simulink model "Drone_PID_rev5_Manual_PID_RL"  (R2021b)
settings: Solver=ode5  StartTime=0.0  StopTime=60  FixedStep=1e-2  RelTol=1e-3
values from neighbouring files (symbols this model uses):
  g = robot.env.g    [A_Main.m]
  Kf = robot.aero.Kthrust    [A_Main.m]
  Km = robot.aero.Ktorque    [A_Main.m]
  L = robot.geom.L    [A_Main.m]
  mass = robot.geom.mass*(0.40*rand()-0.20+1)    [A_Main.m]
  maxRPM = robot.rotor.rpm    [A_Main.m]
  T = [Kf                              Kf                             Kf                             Kf ... (first row only)    [A_Main.m]
  Tinv = inv(T)    [A_Main.m]
  Wmax = maxRPM*2*pi/60    [A_Main.m]
undefined symbols (not defined in the file or in its folder): DiscIntNeverNeededParam, sigbuilder_block
libraries: simulink x16, aerolibconvert2 x13, rllib x4, shared6dof x1
settings Model: Creator=Hassan  LastModifiedBy=Hassan
settings SolverCC: AlgebraicLoopSolver=TrustRegion
settings DebuggingCC: ArithmeticOperatorsInVariantConditions=warning
settings SFSimCC: CustomCodeUndefinedFunction=UseInterfaceOnly
settings CodeAppCC: StateflowObjectComments=on

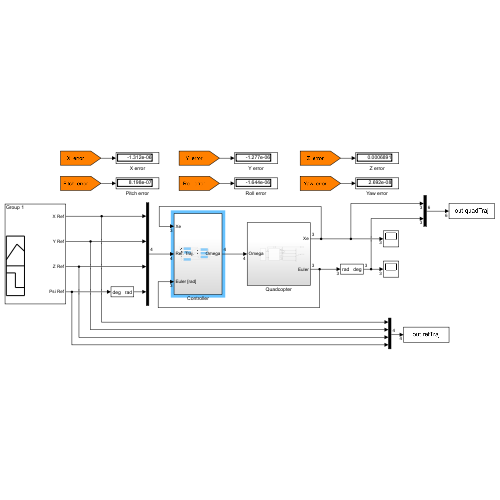
[thumbnail: Simulink's stored preview of the top-level diagram]
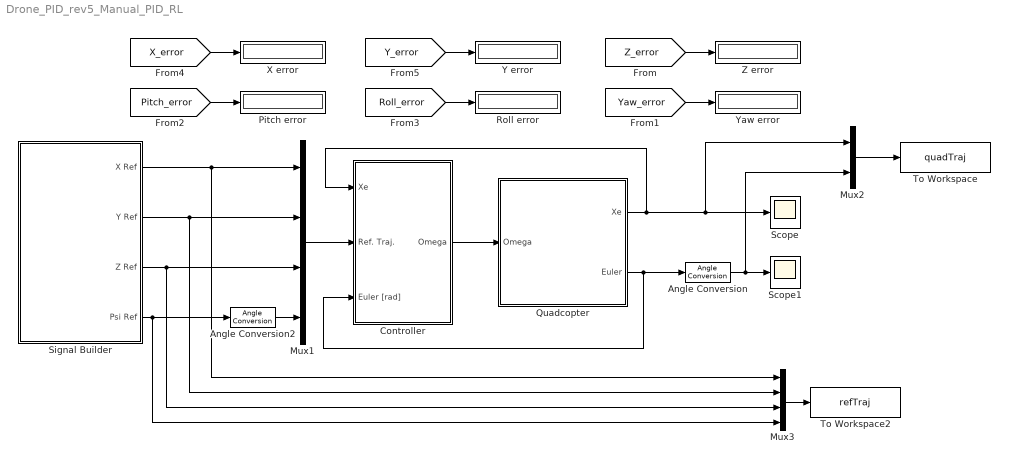
== system Drone_PID_rev5_Manual_PID_RL ==
  Angle Conversion : aerolibconvert2/Angle Conversion  IU=rad  OU=deg
  Angle Conversion2 : aerolibconvert2/Angle Conversion  IU=deg  OU=rad
  Controller : Subsystem
  Mux1 : Mux
  Mux2 : Mux  Inputs=2
  Mux3 : Mux
  Pitch error : Display
  Quadcopter : Subsystem
  Roll error : Display
  Scope : Scope
  Scope1 : Scope
  Signal Builder : Subsystem  Tag=STV Subsys  LoadFcn=sigbuilder_block('load');  StartFcn=sigbuilder_block('start');  StopFcn=sigbuilder_block('stop');  ClipboardFcn=sigbuilder_block('clipboard');  mask(Sigbuilder block){tuvar=[0:10]}
      mask help: Simulink:masks:SigbuilderBlock_MD
      mask init:
      | if ~strcmp(get_param(bdroot(gcbh),'SimulationStatus'),'stopped') tuvar = sigbuilder_block('maskInit'); end
      settings: CopyFcn=sigbuilder_block('copy');  DeleteFcn=sigbuilder_block('delete');  ModelCloseFcn=sigbuilder_block('modelClose');  PreSaveFcn=sigbuilder_block('preSave');  PauseFcn=sigbuilder_block('pause');  ContinueFcn=sigbuilder_block('continue');  NameChangeFcn=sigbuilder_block('namechange');  OpenFcn=sigbuilder_block('open',[379.8 118.8 550.8 400.2 ]);  CloseFcn=sigbuilder_block('close');
      mask Display: plot(0, 0, 100, 100,[2, 2, 32, 32, 2], [68, 8, 8, 68, 68],[32, 2], [38, 38], [32, 19, 2],[53, 60, 44], [32, 17, 17, 2],[16, 16, 31, 31]);txt = getActiveGroup(gcbh);text(2, 100, txt,'verticalAlignment', 'top');
  To Workspace : ToWorkspace  VariableName=quadTraj  SaveFormat=Timeseries  SampleTime=-1
  To Workspace2 : ToWorkspace  VariableName=refTraj  SaveFormat=Timeseries  SampleTime=-1
  X error : Display
  Y error : Display
  Yaw error : Display
  Z error : Display
  wires:
  [Z_error] -> Z error/1
  Angle Conversion/1 -> Mux2/2, Scope1/1
  [Yaw_error] -> Yaw error/1
  [Pitch_error] -> Pitch error/1
  [Roll_error] -> Roll error/1
  Quadcopter/2(Euler) -> Controller/3(Euler [rad]), Angle Conversion/1
  Quadcopter/1(Xe) -> Mux2/1, Scope/1, Controller/1(Xe)
  Controller/1(Omega) -> Quadcopter/1(Omega)
  [Y_error] -> Y error/1
  [X_error] -> X error/1
  Mux1/1 -> Controller/2("Ref. Traj. ")
  Angle Conversion2/1 -> Mux1/4
  Mux3/1 -> To Workspace2/1
  Mux2/1 -> To Workspace/1
  Signal Builder/1(X Ref) -> Mux3/1, Mux1/1
  Signal Builder/2(Y Ref) -> Mux3/2, Mux1/2
  Signal Builder/3(Z Ref) -> Mux3/3, Mux1/3
  Signal Builder/4(Psi Ref) -> Mux3/4, Angle Conversion2/1

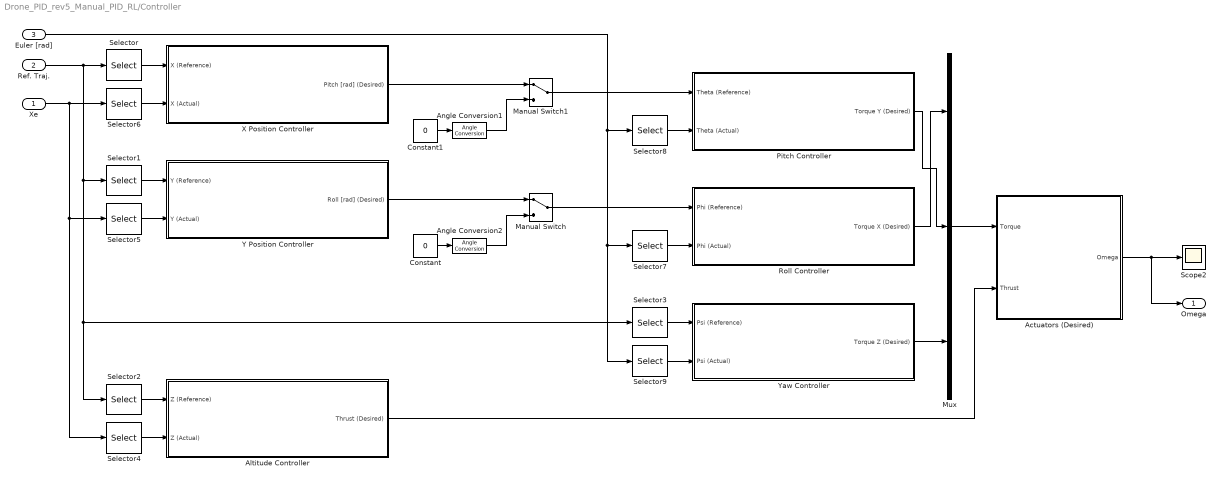
== system Drone_PID_rev5_Manual_PID_RL/Controller ==
  Xe : Inport
  "Ref. Traj. " : Inport  Port=2
  Euler [rad] : Inport  Port=3
  Actuators (Desired) : Subsystem
  Altitude Controller : Subsystem
  Angle Conversion1 : aerolibconvert2/Angle Conversion  IU=deg  OU=rad
  Angle Conversion2 : aerolibconvert2/Angle Conversion  IU=deg  OU=rad
  Constant : Constant  Value=0
  Constant1 : Constant  Value=0
  Manual Switch : ManualSwitch
  Manual Switch1 : ManualSwitch
  Mux : Mux  Inputs=3
  Pitch Controller : Subsystem
  Roll Controller : Subsystem
  Scope2 : Scope
  Selector : Selector  InputPortWidth=4  IndexOptions=Index vector (dialog)  Indices=[1]  OutputSizes=1
  Selector1 : Selector  InputPortWidth=4  IndexOptions=Index vector (dialog)  Indices=[2]  OutputSizes=1
  Selector2 : Selector  InputPortWidth=4  IndexOptions=Index vector (dialog)  Indices=[3]  OutputSizes=1
  Selector3 : Selector  InputPortWidth=4  IndexOptions=Index vector (dialog)  Indices=[4]  OutputSizes=1
  Selector4 : Selector  InputPortWidth=3  IndexOptions=Index vector (dialog)  Indices=[3]  OutputSizes=1
  Selector5 : Selector  InputPortWidth=3  IndexOptions=Index vector (dialog)  Indices=[2]  OutputSizes=1
  Selector6 : Selector  InputPortWidth=3  IndexOptions=Index vector (dialog)  Indices=[1]  OutputSizes=1
  Selector7 : Selector  InputPortWidth=3  IndexOptions=Index vector (dialog)  Indices=[1]  OutputSizes=1
  Selector8 : Selector  InputPortWidth=3  IndexOptions=Index vector (dialog)  Indices=[2]  OutputSizes=1
  Selector9 : Selector  InputPortWidth=3  IndexOptions=Index vector (dialog)  Indices=[3]  OutputSizes=1
  X Position Controller : Subsystem
  Y Position Controller : Subsystem
  Yaw Controller : Subsystem
  Omega : Outport  VectorParamsAs1DForOutWhenUnconnected=off
  wires:
  Actuators (Desired)/1(Omega) -> Scope2/1, Omega/1
  Altitude Controller/1(Thrust (Desired)) -> Actuators (Desired)/2(Thrust)
  Mux/1 -> Actuators (Desired)/1(Torque)
  Xe/1 -> Selector4/1, Selector5/1, Selector6/1
  Selector3/1 -> Yaw Controller/1(Psi (Reference))
  Selector/1 -> X Position Controller/1(X (Reference))
  Selector1/1 -> Y Position Controller/1(Y (Reference))
  Selector2/1 -> Altitude Controller/1(Z (Reference))
  "Ref. Traj. "/1 -> Selector2/1, Selector3/1, Selector1/1, Selector/1
  Selector4/1 -> Altitude Controller/2(Z (Actual))
  Selector5/1 -> Y Position Controller/2(Y (Actual))
  Selector6/1 -> X Position Controller/2(X (Actual))
  Selector7/1 -> Roll Controller/2(Phi (Actual))
  Selector8/1 -> Pitch Controller/2(Theta (Actual))
  Selector9/1 -> Yaw Controller/2(Psi (Actual))
  Euler [rad]/1 -> Selector9/1, Selector7/1, Selector8/1
  Yaw Controller/1(Torque Z (Desired)) -> Mux/3
  Roll Controller/1(Torque X (Desired)) -> Mux/1
  Constant/1 -> Angle Conversion2/1
  Angle Conversion2/1 -> Manual Switch/2
  Manual Switch/1 -> Roll Controller/1(Phi (Reference))
  Y Position Controller/1(Roll [rad] (Desired)) -> Manual Switch/1
  Pitch Controller/1(Torque Y (Desired)) -> Mux/2
  Manual Switch1/1 -> Pitch Controller/1(Theta (Reference))
  X Position Controller/1(Pitch [rad] (Desired)) -> Manual Switch1/1
  Constant1/1 -> Angle Conversion1/1
  Angle Conversion1/1 -> Manual Switch1/2

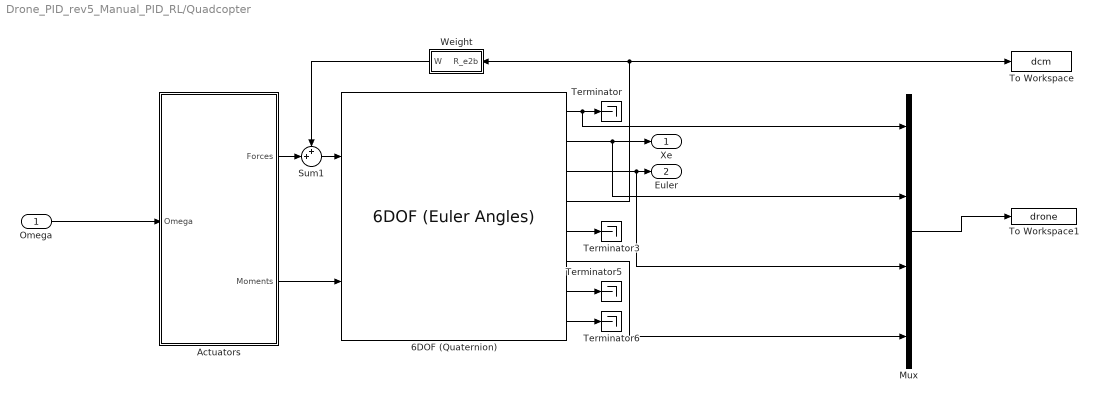
== system Drone_PID_rev5_Manual_PID_RL/Quadcopter ==
  Omega : Inport
  6DOF (Quaternion) : shared6dof/6DOF (Euler Angles)  units=Metric (MKS)  mtype=Fixed  rep=Quaternion  xme_0=pos_I_init  Vm_0=vel_B_init  eul_0=euler_I_init  pm_0=angvel_B_init  mass_0=mass  mass_e=0.5  mass_f=2.0  inertia=J  inertia_e=eye(3)  inertia_f=2*eye(3)  k_quat=1.0  vre_flag=on  abi_flag=off  aMode=aMode  xme_statename=''  Vm_statename=''  eul_statename=''  quat_statename=''  pm_statename=''  mass_statename=''
      settings: SourceProductBaseCode=AE,PW,DR,MT,UV,VE
  Actuators : Subsystem
  Mux : Mux
  Sum1 : Sum  Inputs=++|
  Terminator{,3,5..6} (4 alike) : Terminator
  To Workspace : ToWorkspace  VariableName=dcm  SaveFormat=Timeseries  SampleTime=-1
  To Workspace1 : ToWorkspace  VariableName=drone  SaveFormat=Timeseries  SampleTime=-1
  Weight : Subsystem
      mask Display: disp('Weight')
  Xe : Outport  VectorParamsAs1DForOutWhenUnconnected=off
  Euler : Outport  Port=2  VectorParamsAs1DForOutWhenUnconnected=off
  wires:
  6DOF (Quaternion)/1 -> Mux/1, Terminator/1
  6DOF (Quaternion)/8 -> Terminator6/1
  Actuators/1(Forces) -> Sum1/2
  Actuators/2(Moments) -> 6DOF (Quaternion)/2
  6DOF (Quaternion)/7 -> Terminator5/1
  6DOF (Quaternion)/4 -> Weight/1(R_e2b), To Workspace/1
  6DOF (Quaternion)/5 -> Terminator3/1
  6DOF (Quaternion)/6 -> Mux/4
  6DOF (Quaternion)/3 -> Euler/1, Mux/3
  6DOF (Quaternion)/2 -> Mux/2, Xe/1
  Omega/1 -> Actuators/1(Omega)
  Weight/1(W) -> Sum1/1
  Sum1/1 -> 6DOF (Quaternion)/1
  Mux/1 -> To Workspace1/1

== system Drone_PID_rev5_Manual_PID_RL/Signal Builder ==
  Demux : Demux  Tag=STV Demux
      settings: DisplayOption=none
  FromWs : FromWorkspace  Tag=STV FromWs  VariableName=tuvar
      SigBuilderData=|
      | common.afterFinalStr = 'Extrapolate'
      | common.sampleTime = 0
      | dataSet.timeRange = [0 60]
      | dataSet.name = 'Group 1'
      | sbobj.Groups.Name = 'Group 1'
      | sbobj.Groups.Signals(1).Name = 'X Ref'
      | sbobj.Groups.Signals(1).XData = [0 0.01 0.02 0.03 0.04 0.05 0.06 0.07 0.08 0.09 0.1 0.11 ... (6001 elements, 1x6001)]
      | sbobj.Groups.Signals(1).YData = [0 0 0 0 0 0 0 0 0 0 0 0 ... (6001 elements, 1x6001)]
      | sbobj.Groups.Signals(2).Name = 'Y Ref'
      | sbobj.Groups.Signals(2).XData = [0 0.01 0.02 0.03 0.04 0.05 0.06 0.07 0.08 0.09 0.1 0.11 ... (6001 elements, 1x6001)]
      | sbobj.Groups.Signals(2).YData = [0 0 0 0 0 0 0 0 0 0 0 0 ... (6001 elements, 1x6001)]
      | sbobj.Groups.Signals(3).Name = 'Z Ref'
      | sbobj.Groups.Signals(3).XData = [0 0.01 0.02 0.03 0.04 0.05 0.06 0.07 0.08 0.09 0.1 0.11 ... (6001 elements, 1x6001)]
      | sbobj.Groups.Signals(3).YData = [0 0 0 0 0 0 0 0 0 0 0 0 ... (6001 elements, 1x6001)]
      | sbobj.Groups.Signals(4).Name = 'Psi Ref'
      | sbobj.Groups.Signals(4).XData = [0 60]
      | sbobj.Groups.Signals(4).YData = [0 0]
      | sbobj.Groups.TimeRange = [0 60]
  X Ref : Outport  Tag=STV Outport
  Y Ref : Outport  Tag=STV Outport  Port=2
  Z Ref : Outport  Tag=STV Outport  Port=3
  Psi Ref : Outport  Tag=STV Outport  Port=4
  wires:
  FromWs/1 -> Demux/1
  Demux/1 -> X Ref/1
  Demux/2 -> Y Ref/1
  Demux/3 -> Z Ref/1
  Demux/4 -> Psi Ref/1

== system Drone_PID_rev5_Manual_PID_RL/Controller/Actuators (Desired) ==
  Torque : Inport
  Thrust : Inport  Port=2
  Gain : Gain  Gain=Tinv  Multiplication=Matrix(K*u)
  Limit Omega (rad/sec) due to Motor Constraints : Saturate  UpperLimit=Wmax  LowerLimit=0
  Mux : Mux  Inputs=2
  Sqrt : Sqrt  SaturateOnIntegerOverflow=on
  Omega : Outport  VectorParamsAs1DForOutWhenUnconnected=off
  wires:
  Torque/1 -> Mux/2
  Thrust/1 -> Mux/1
  Limit Omega (rad/sec) due to Motor Constraints/1 -> Omega/1
  Sqrt/1 -> Limit Omega (rad/sec) due to Motor Constraints/1
  Gain/1 -> Sqrt/1
  Mux/1 -> Gain/1

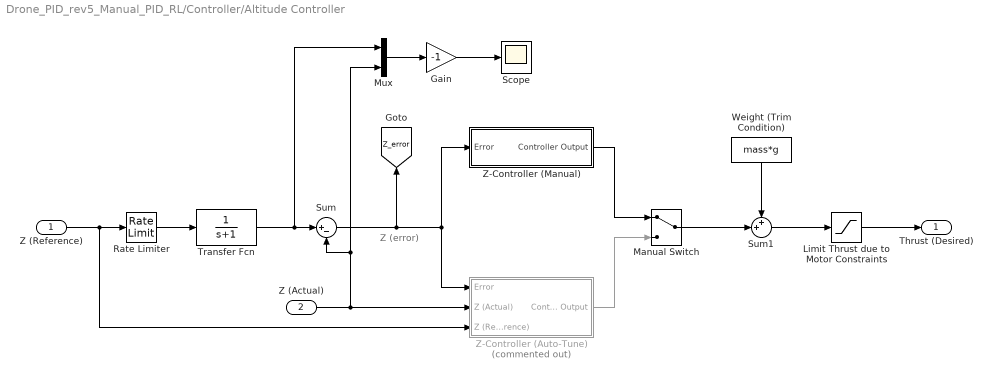
== system Drone_PID_rev5_Manual_PID_RL/Controller/Altitude Controller ==
  note: Z (error)
  Z (Reference) : Inport
  Z (Actual) : Inport  Port=2
  Gain : Gain  Gain=-1
  Limit Thrust due to Motor Constraints : Saturate  UpperLimit=4*Kf*(Wmax^2)  LowerLimit=0
  Manual Switch : ManualSwitch
  Mux : Mux  Inputs=2
  Rate Limiter : RateLimiter  RisingSlewLimit=2  FallingSlewLimit=-2  SampleTimeMode=inherited
  Scope : Scope
  Sum : Sum  Inputs=|+-
  Sum1 : Sum  Inputs=++|
  Transfer Fcn : TransferFcn  Denominator=[1 1]
  Weight (Trim Condition) : Constant  Value=mass*g
  Z-Controller (Auto-Tune) : Subsystem  Commented=on
  Z-Controller (Manual) : Subsystem
  Thrust (Desired) : Outport  VectorParamsAs1DForOutWhenUnconnected=off
  tag scope: Z_error=global
  wires:
  Weight (Trim Condition)/1 -> Sum1/1
  Sum/1 -> [Z_error], Z-Controller (Auto-Tune)/1(Error), Z-Controller (Manual)/1(Error)
  Sum1/1 -> Limit Thrust due to Motor Constraints/1
  Limit Thrust due to Motor Constraints/1 -> Thrust (Desired)/1
  Mux/1 -> Gain/1
  Z (Reference)/1 -> Z-Controller (Auto-Tune)/3(Z (Reference)), Rate Limiter/1
  Z (Actual)/1 -> Sum/2, Mux/2, Z-Controller (Auto-Tune)/2(Z (Actual))
  Gain/1 -> Scope/1
  Transfer Fcn/1 -> Mux/1, Sum/1
  Rate Limiter/1 -> Transfer Fcn/1
  Manual Switch/1 -> Sum1/2
  Z-Controller (Manual)/1(Controller Output) -> Manual Switch/1
  Z-Controller (Auto-Tune)/1(Controller Output) -> Manual Switch/2

== system Drone_PID_rev5_Manual_PID_RL/Controller/Pitch Controller ==
  note: Theta (Error)
  Theta (Reference) : Inport
  Theta (Actual) : Inport  Port=2
  Angle Conversion : aerolibconvert2/Angle Conversion  IU=rad  OU=deg
  Limit Pitch Torque due to Motor Constraints : Saturate  UpperLimit=(Kf*(maxRPM*(2*pi)/60)^2)*L  LowerLimit=-(Kf*(maxRPM*(2*pi)/60)^2)*L
  Mux : Mux  Inputs=2
  Pitch-Controller : Subsystem
  Scope : Scope
  Sum2 : Sum  Inputs=|+-
  Torque Y (Desired) : Outport  VectorParamsAs1DForOutWhenUnconnected=off
  tag scope: Pitch_error=global
  wires:
  Sum2/1 -> [Pitch_error], Pitch-Controller/1(Error)
  Pitch-Controller/1(Controller Output) -> Limit Pitch Torque due to Motor Constraints/1
  Limit Pitch Torque due to Motor Constraints/1 -> Torque Y (Desired)/1
  Angle Conversion/1 -> Scope/1
  Mux/1 -> Angle Conversion/1
  Theta (Actual)/1 -> Mux/2, Sum2/2
  Theta (Reference)/1 -> Mux/1, Sum2/1

== system Drone_PID_rev5_Manual_PID_RL/Controller/Roll Controller ==
  note: Phi (Error)
  Phi (Reference) : Inport
  Phi (Actual) : Inport  Port=2
  Angle Conversion : aerolibconvert2/Angle Conversion  IU=rad  OU=deg
  Limit Roll Torque due to Motor Constraints : Saturate  UpperLimit=Kf*(Wmax^2)*L  LowerLimit=-Kf*(Wmax^2)*L
  Manual Switch : ManualSwitch
  Mux : Mux  Inputs=2
  Roll-Controller : Subsystem
  Roll-Controller (Auto-Tune) : Subsystem  Commented=on
  Scope : Scope
  Sum2 : Sum  Inputs=|+-
  Torque X (Desired) : Outport  VectorParamsAs1DForOutWhenUnconnected=off
  tag scope: Roll_error=global
  wires:
  Phi (Reference)/1 -> Roll-Controller (Auto-Tune)/3(Roll (Reference)), Sum2/1, Mux/1
  Sum2/1 -> Roll-Controller (Auto-Tune)/1(Error), [Roll_error], Roll-Controller/1(Error)
  Limit Roll Torque due to Motor Constraints/1 -> Torque X (Desired)/1
  Mux/1 -> Angle Conversion/1
  Phi (Actual)/1 -> Mux/2, Sum2/2, Roll-Controller (Auto-Tune)/2(Roll (Actual))
  Angle Conversion/1 -> Scope/1
  Manual Switch/1 -> Limit Roll Torque due to Motor Constraints/1
  Roll-Controller/1(Controller Output) -> Manual Switch/1
  Roll-Controller (Auto-Tune)/1(Controller Output) -> Manual Switch/2

== system Drone_PID_rev5_Manual_PID_RL/Controller/X Position Controller ==
  note: X (Error)
  X (Reference) : Inport
  X (Actual) : Inport  Port=2
  Limit Pitch Ref : Saturate  UpperLimit=25*pi/180  LowerLimit=-25*pi/180
  Mux : Mux  Inputs=2
  Rate Limiter : RateLimiter  RisingSlewLimit=3  FallingSlewLimit=-3  SampleTimeMode=inherited
  Scope : Scope
  Sum2 : Sum  Inputs=|+-
  Transfer Fcn : TransferFcn  Numerator=[2]  Denominator=[1 2]
  X-Controller : Subsystem
  Pitch [rad] (Desired) : Outport  VectorParamsAs1DForOutWhenUnconnected=off
  tag scope: X_error=global
  wires:
  Sum2/1 -> [X_error], X-Controller/1(Error)
  X-Controller/1(Controller Output) -> Limit Pitch Ref/1
  Mux/1 -> Scope/1
  X (Reference)/1 -> Rate Limiter/1
  X (Actual)/1 -> Mux/2, Sum2/2
  Limit Pitch Ref/1 -> Pitch [rad] (Desired)/1
  Transfer Fcn/1 -> Mux/1, Sum2/1
  Rate Limiter/1 -> Transfer Fcn/1

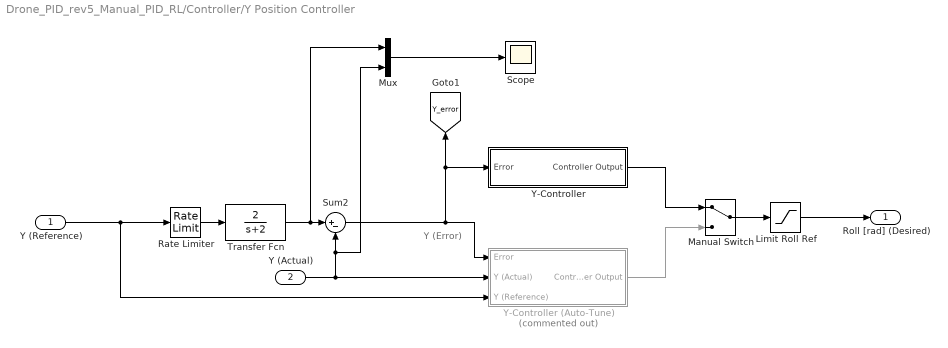
== system Drone_PID_rev5_Manual_PID_RL/Controller/Y Position Controller ==
  note: Y (Error)
  Y (Reference) : Inport
  Y (Actual) : Inport  Port=2
  Limit Roll Ref : Saturate  UpperLimit=25*pi/180  LowerLimit=-25*pi/180
  Manual Switch : ManualSwitch
  Mux : Mux  Inputs=2
  Rate Limiter : RateLimiter  RisingSlewLimit=3  FallingSlewLimit=-3  SampleTimeMode=inherited
  Scope : Scope
  Sum2 : Sum  Inputs=|+-
  Transfer Fcn : TransferFcn  Numerator=[2]  Denominator=[1 2]
  Y-Controller : Subsystem
  Y-Controller (Auto-Tune) : Subsystem  Commented=on
  Roll [rad] (Desired) : Outport  VectorParamsAs1DForOutWhenUnconnected=off
  tag scope: Y_error=global
  wires:
  Y (Reference)/1 -> Y-Controller (Auto-Tune)/3(Y (Reference)), Rate Limiter/1
  Sum2/1 -> Y-Controller (Auto-Tune)/1(Error), Y-Controller/1(Error), [Y_error]
  Y (Actual)/1 -> Y-Controller (Auto-Tune)/2(Y (Actual)), Mux/2, Sum2/2
  Mux/1 -> Scope/1
  Limit Roll Ref/1 -> Roll [rad] (Desired)/1
  Rate Limiter/1 -> Transfer Fcn/1
  Transfer Fcn/1 -> Mux/1, Sum2/1
  Manual Switch/1 -> Limit Roll Ref/1
  Y-Controller/1(Controller Output) -> Manual Switch/1
  Y-Controller (Auto-Tune)/1(Controller Output) -> Manual Switch/2

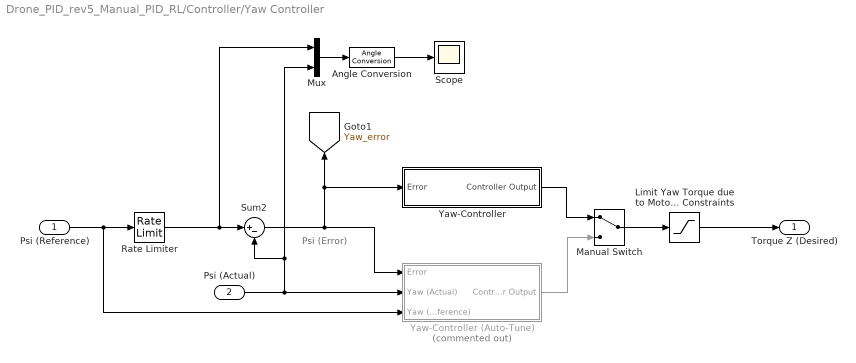
== system Drone_PID_rev5_Manual_PID_RL/Controller/Yaw Controller ==
  note: Psi (Error)
  Psi (Reference) : Inport
  Psi (Actual) : Inport  Port=2
  Angle Conversion : aerolibconvert2/Angle Conversion  IU=rad  OU=deg
  Limit Yaw Torque due to Motor Constraints : Saturate  UpperLimit=(Km*(maxRPM*(2*pi)/60)^2)  LowerLimit=-(Km*(maxRPM*(2*pi)/60)^2)
  Manual Switch : ManualSwitch
  Mux : Mux  Inputs=2
  Rate Limiter : RateLimiter  RisingSlewLimit=10*pi/180  FallingSlewLimit=-10*pi/180  SampleTimeMode=inherited
  Scope : Scope
  Sum2 : Sum  Inputs=|+-
  Yaw-Controller : Subsystem
  Yaw-Controller (Auto-Tune) : Subsystem  Commented=on
  Torque Z (Desired) : Outport  VectorParamsAs1DForOutWhenUnconnected=off
  tag scope: Yaw_error=global
  wires:
  Limit Yaw Torque due to Motor Constraints/1 -> Torque Z (Desired)/1
  Sum2/1 -> Yaw-Controller (Auto-Tune)/1(Error), [Yaw_error], Yaw-Controller/1(Error)
  Angle Conversion/1 -> Scope/1
  Mux/1 -> Angle Conversion/1
  Psi (Actual)/1 -> Sum2/2, Mux/2, Yaw-Controller (Auto-Tune)/2(Yaw (Actual))
  Psi (Reference)/1 -> Yaw-Controller (Auto-Tune)/3(Yaw (Reference)), Rate Limiter/1
  Rate Limiter/1 -> Mux/1, Sum2/1
  Manual Switch/1 -> Limit Yaw Torque due to Motor Constraints/1
  Yaw-Controller/1(Controller Output) -> Manual Switch/1
  Yaw-Controller (Auto-Tune)/1(Controller Output) -> Manual Switch/2

== system Drone_PID_rev5_Manual_PID_RL/Quadcopter/Actuators ==
  Omega : Inport
  Constant : Constant  Value=0
  Demux : Demux  Outputs=[1 3]
  Gain : Gain  Gain=T  Multiplication=Matrix(K*u)
  Gain1 : Gain  Gain=-1
  Mux : Mux  Inputs=3
  Product : Product
  Forces : Outport  VectorParamsAs1DForOutWhenUnconnected=off
  Moments : Outport  Port=2  VectorParamsAs1DForOutWhenUnconnected=off
  wires:
  Gain/1 -> Demux/1
  Demux/2 -> Moments/1
  Demux/1 -> Gain1/1
  Constant/1 -> Mux/1, Mux/2
  Mux/1 -> Forces/1
  Omega/1 -> Product/2, Product/1
  Product/1 -> Gain/1
  Gain1/1 -> Mux/3

== system Drone_PID_rev5_Manual_PID_RL/Quadcopter/Weight ==
  R_e2b : Inport
  Constant1 : Constant  Value=[0 0 g]
  Product : Product  Multiplication=Matrix(*)
  mass : Gain  Gain=mass
  W : Outport  VectorParamsAs1DForOutWhenUnconnected=off
  wires:
  Product/1 -> mass/1
  Constant1/1 -> Product/2
  R_e2b/1 -> Product/1
  mass/1 -> W/1

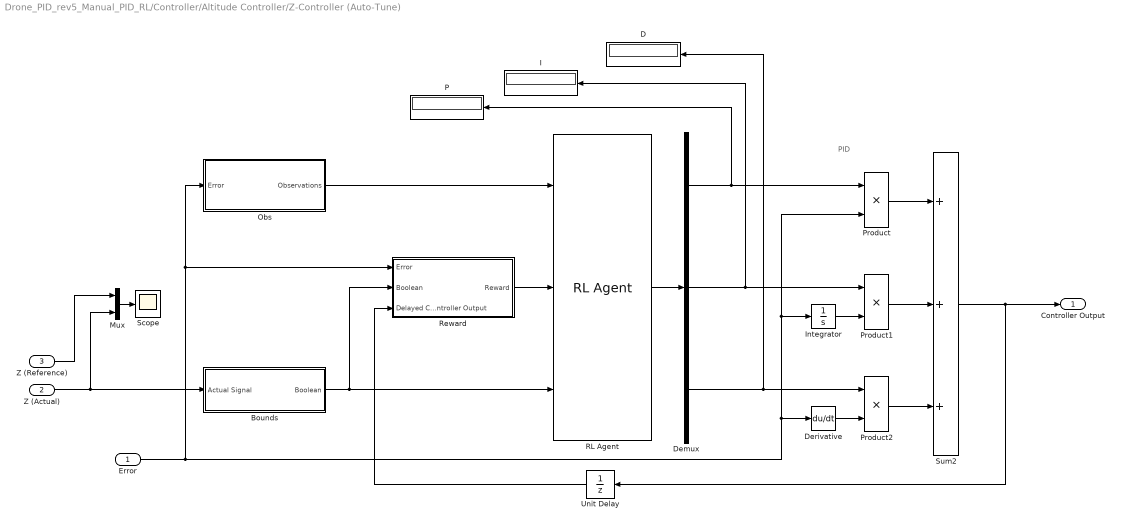
== system Drone_PID_rev5_Manual_PID_RL/Controller/Altitude Controller/Z-Controller (Auto-Tune) ==
  note: PID
  Error : Inport
  Z (Actual) : Inport  Port=2
  Z (Reference) : Inport  Port=3
  Bounds : Subsystem
  D : Display
  Demux : Demux  Outputs=3
  Derivative : Derivative
  I : Display
  Integrator : Integrator
  Mux : Mux  Inputs=2
  Obs : Subsystem
  P : Display
  Product : Product
  Product1 : Product
  Product2 : Product
  RL Agent : rllib/RL Agent  Agent=agent  ExternalActionAsInput=off  ProvideCumRwd=off  TreatAsDirectFeedthrough=on
  Reward : Subsystem
  Scope : Scope
  Sum2 : Sum  Inputs=+++
  Unit Delay : UnitDelay  SampleTime=-1  HasFrameUpgradeWarning=on
  Controller Output : Outport
  wires:
  Demux/2 -> Product1/1, I/1
  Sum2/1 -> Unit Delay/1, Controller Output/1
  Product2/1 -> Sum2/3
  Derivative/1 -> Product2/2
  Product1/1 -> Sum2/2
  Error/1 -> Product/2, Integrator/1, Derivative/1, Reward/1(Error), Obs/1(Error)
  Product/1 -> Sum2/1
  Integrator/1 -> Product1/2
  RL Agent/1 -> Demux/1
  Demux/1 -> Product/1, P/1
  Demux/3 -> Product2/1, D/1
  Obs/1(Observations) -> RL Agent/1
  Z (Actual)/1 -> Mux/2, Bounds/1(Actual Signal)
  Bounds/1(Boolean) -> RL Agent/3, Reward/2(Boolean)
  Unit Delay/1 -> Reward/3(Delayed Controller Output)
  Reward/1(Reward) -> RL Agent/2
  Mux/1 -> Scope/1
  Z (Reference)/1 -> Mux/1

== system Drone_PID_rev5_Manual_PID_RL/Controller/Altitude Controller/Z-Controller (Manual) ==
  Error : Inport
  D : Constant  Value=-2.617
  Derivative : Derivative
  I : Constant  Value=0
  Integrator : Integrator
  P : Constant  Value=-3.028
  Product : Product
  Product1 : Product
  Product2 : Product
  Sum2 : Sum  Inputs=+++
  Controller Output : Outport
  wires:
  I/1 -> Product1/1
  Sum2/1 -> Controller Output/1
  Product2/1 -> Sum2/3
  Derivative/1 -> Product2/2
  Product1/1 -> Sum2/2
  Error/1 -> Product/2, Derivative/1, Integrator/1
  P/1 -> Product/1
  Product/1 -> Sum2/1
  Integrator/1 -> Product1/2
  D/1 -> Product2/1

== system Drone_PID_rev5_Manual_PID_RL/Controller/Pitch Controller/Pitch-Controller ==
  Error : Inport
  D : Constant  Value=0.003858
  Derivative : Derivative
  I : Constant  Value=0.0006933
  Integrator : Integrator
  P : Constant  Value=0.006892
  Product : Product
  Product1 : Product
  Product2 : Product
  Sum2 : Sum  Inputs=+++
  Controller Output : Outport
  wires:
  I/1 -> Product1/1
  Sum2/1 -> Controller Output/1
  Product2/1 -> Sum2/3
  Derivative/1 -> Product2/2
  Product1/1 -> Sum2/2
  Error/1 -> Product/2, Derivative/1, Integrator/1
  P/1 -> Product/1
  Product/1 -> Sum2/1
  Integrator/1 -> Product1/2
  D/1 -> Product2/1

== system Drone_PID_rev5_Manual_PID_RL/Controller/Roll Controller/Roll-Controller ==
  Error : Inport
  D : Constant  Value=0.003858
  Derivative : Derivative
  I : Constant  Value=0.0006933
  Integrator : Integrator
  P : Constant  Value=0.006829
  Product : Product
  Product1 : Product
  Product2 : Product
  Sum2 : Sum  Inputs=+++
  Controller Output : Outport
  wires:
  I/1 -> Product1/1
  Sum2/1 -> Controller Output/1
  Product2/1 -> Sum2/3
  Derivative/1 -> Product2/2
  Product1/1 -> Sum2/2
  Error/1 -> Product/2, Derivative/1, Integrator/1
  P/1 -> Product/1
  Product/1 -> Sum2/1
  Integrator/1 -> Product1/2
  D/1 -> Product2/1

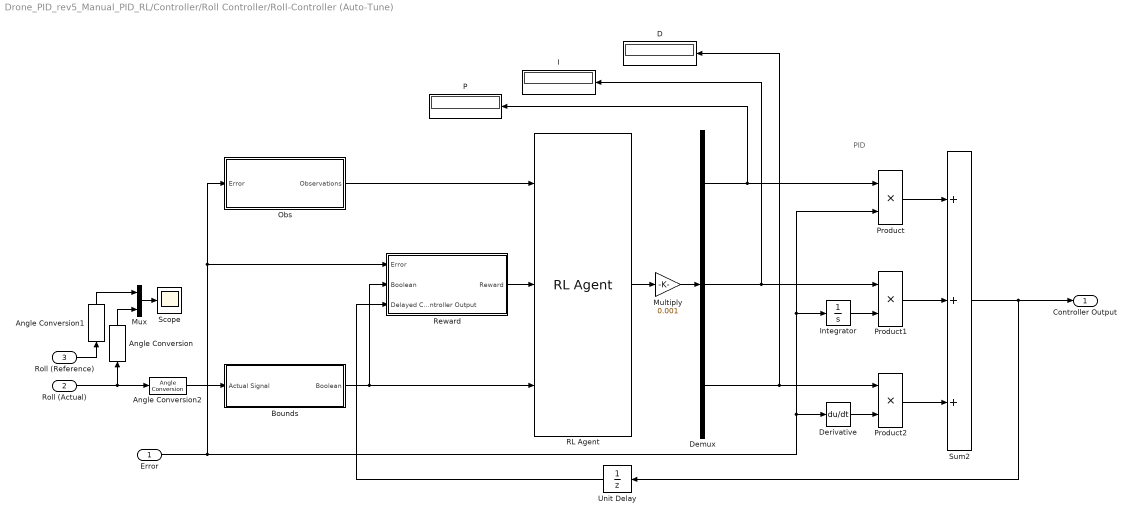
== system Drone_PID_rev5_Manual_PID_RL/Controller/Roll Controller/Roll-Controller (Auto-Tune) ==
  note: PID
  Error : Inport
  Roll (Actual) : Inport  Port=2
  Roll (Reference) : Inport  Port=3
  Angle Conversion : aerolibconvert2/Angle Conversion  IU=rad  OU=deg
  Angle Conversion1 : aerolibconvert2/Angle Conversion  IU=rad  OU=deg
  Angle Conversion2 : aerolibconvert2/Angle Conversion  IU=rad  OU=deg
  Bounds : Subsystem
  D : Display
  Demux : Demux  Outputs=3
  Derivative : Derivative
  I : Display
  Integrator : Integrator
  Multiply : Gain  Gain=0.001
  Mux : Mux  Inputs=2
  Obs : Subsystem
  P : Display
  Product : Product
  Product1 : Product
  Product2 : Product
  RL Agent : rllib/RL Agent  Agent=agent  ExternalActionAsInput=off  ProvideCumRwd=off  TreatAsDirectFeedthrough=on
  Reward : Subsystem
  Scope : Scope
  Sum2 : Sum  Inputs=+++
  Unit Delay : UnitDelay  SampleTime=-1  HasFrameUpgradeWarning=on
  Controller Output : Outport
  wires:
  Demux/2 -> Product1/1, I/1
  Sum2/1 -> Unit Delay/1, Controller Output/1
  Product2/1 -> Sum2/3
  Derivative/1 -> Product2/2
  Product1/1 -> Sum2/2
  Error/1 -> Product/2, Integrator/1, Derivative/1, Obs/1(Error), Reward/1(Error)
  Product/1 -> Sum2/1
  Integrator/1 -> Product1/2
  Demux/1 -> Product/1, P/1
  Demux/3 -> Product2/1, D/1
  Obs/1(Observations) -> RL Agent/1
  Roll (Actual)/1 -> Angle Conversion/1, Angle Conversion2/1
  Bounds/1(Boolean) -> RL Agent/3, Reward/2(Boolean)
  Unit Delay/1 -> Reward/3(Delayed Controller Output)
  Reward/1(Reward) -> RL Agent/2
  Mux/1 -> Scope/1
  Roll (Reference)/1 -> Angle Conversion1/1
  Angle Conversion/1 -> Mux/2
  Angle Conversion1/1 -> Mux/1
  RL Agent/1 -> Multiply/1
  Angle Conversion2/1 -> Bounds/1(Actual Signal)
  Multiply/1 -> Demux/1

== system Drone_PID_rev5_Manual_PID_RL/Controller/X Position Controller/X-Controller ==
  Error : Inport
  D : Constant  Value=-.3552
  Derivative : Derivative
  I : Constant  Value=-.00617
  Integrator : Integrator
  P : Constant  Value=-2.17
  Product : Product
  Product1 : Product
  Product2 : Product
  Sum2 : Sum  Inputs=+++
  Controller Output : Outport
  wires:
  I/1 -> Product1/1
  Sum2/1 -> Controller Output/1
  Product2/1 -> Sum2/3
  Derivative/1 -> Product2/2
  Product1/1 -> Sum2/2
  Error/1 -> Product/2, Derivative/1, Integrator/1
  P/1 -> Product/1
  Product/1 -> Sum2/1
  Integrator/1 -> Product1/2
  D/1 -> Product2/1

== system Drone_PID_rev5_Manual_PID_RL/Controller/Y Position Controller/Y-Controller ==
  Error : Inport
  D : Constant  Value=0.3552
  Derivative : Derivative
  I : Constant  Value=0.00617
  Integrator : Integrator
  P : Constant  Value=2.17
  Product : Product
  Product1 : Product
  Product2 : Product
  Sum2 : Sum  Inputs=+++
  Controller Output : Outport
  wires:
  I/1 -> Product1/1
  Sum2/1 -> Controller Output/1
  Product2/1 -> Sum2/3
  Derivative/1 -> Product2/2
  Product1/1 -> Sum2/2
  Error/1 -> Product/2, Derivative/1, Integrator/1
  P/1 -> Product/1
  Product/1 -> Sum2/1
  Integrator/1 -> Product1/2
  D/1 -> Product2/1

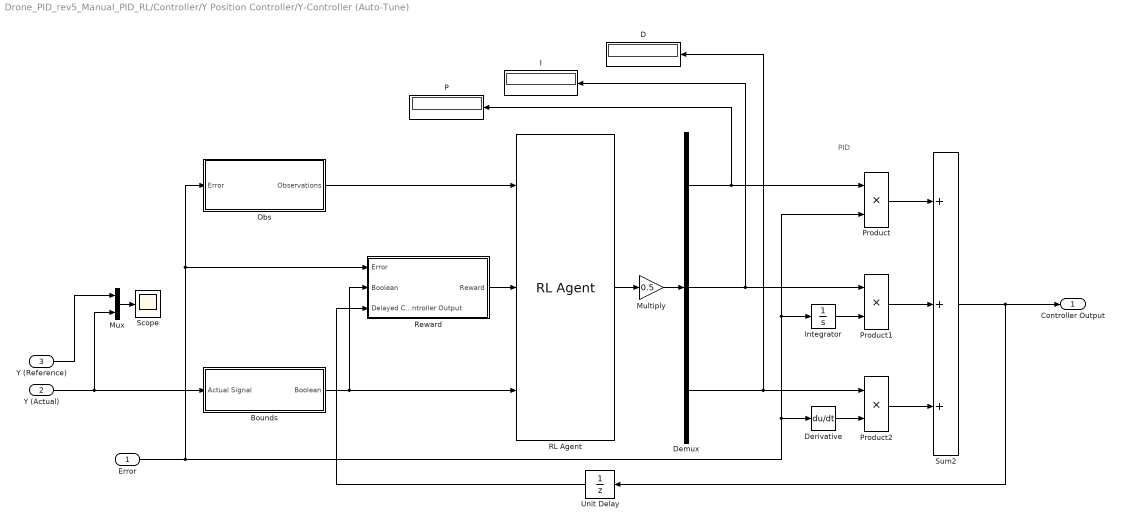
== system Drone_PID_rev5_Manual_PID_RL/Controller/Y Position Controller/Y-Controller (Auto-Tune) ==
  note: PID
  Error : Inport
  Y (Actual) : Inport  Port=2
  Y (Reference) : Inport  Port=3
  Bounds : Subsystem
  D : Display
  Demux : Demux  Outputs=3
  Derivative : Derivative
  I : Display
  Integrator : Integrator
  Multiply : Gain  Gain=0.5
  Mux : Mux  Inputs=2
  Obs : Subsystem
  P : Display
  Product : Product
  Product1 : Product
  Product2 : Product
  RL Agent : rllib/RL Agent  Agent=agent  ExternalActionAsInput=off  ProvideCumRwd=off  TreatAsDirectFeedthrough=on
  Reward : Subsystem
  Scope : Scope
  Sum2 : Sum  Inputs=+++
  Unit Delay : UnitDelay  SampleTime=-1  HasFrameUpgradeWarning=on
  Controller Output : Outport
  wires:
  Demux/2 -> Product1/1, I/1
  Sum2/1 -> Unit Delay/1, Controller Output/1
  Product2/1 -> Sum2/3
  Derivative/1 -> Product2/2
  Product1/1 -> Sum2/2
  Error/1 -> Product/2, Integrator/1, Derivative/1, Obs/1(Error), Reward/1(Error)
  Product/1 -> Sum2/1
  Integrator/1 -> Product1/2
  Demux/1 -> Product/1, P/1
  Demux/3 -> Product2/1, D/1
  Obs/1(Observations) -> RL Agent/1
  Bounds/1(Boolean) -> RL Agent/3, Reward/2(Boolean)
  Unit Delay/1 -> Reward/3(Delayed Controller Output)
  Reward/1(Reward) -> RL Agent/2
  Mux/1 -> Scope/1
  Y (Reference)/1 -> Mux/1
  RL Agent/1 -> Multiply/1
  Y (Actual)/1 -> Bounds/1(Actual Signal), Mux/2
  Multiply/1 -> Demux/1

== system Drone_PID_rev5_Manual_PID_RL/Controller/Yaw Controller/Yaw-Controller ==
  Error : Inport
  D : Constant  Value=0.002166
  Derivative : Derivative
  I : Constant  Value=0.001729
  Integrator : Integrator
  P : Constant  Value=0.00894
  Product : Product
  Product1 : Product
  Product2 : Product
  Sum2 : Sum  Inputs=+++
  Controller Output : Outport
  wires:
  I/1 -> Product1/1
  Sum2/1 -> Controller Output/1
  Product2/1 -> Sum2/3
  Derivative/1 -> Product2/2
  Product1/1 -> Sum2/2
  Error/1 -> Product/2, Derivative/1, Integrator/1
  P/1 -> Product/1
  Product/1 -> Sum2/1
  Integrator/1 -> Product1/2
  D/1 -> Product2/1

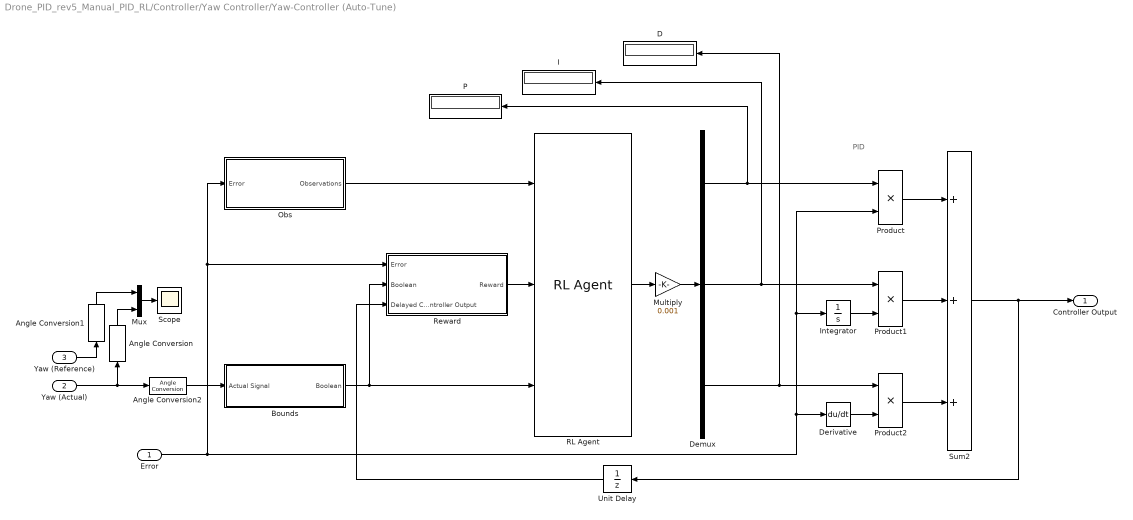
== system Drone_PID_rev5_Manual_PID_RL/Controller/Yaw Controller/Yaw-Controller (Auto-Tune) ==
  note: PID
  Error : Inport
  Yaw (Actual) : Inport  Port=2
  Yaw (Reference) : Inport  Port=3
  Angle Conversion : aerolibconvert2/Angle Conversion  IU=rad  OU=deg
  Angle Conversion1 : aerolibconvert2/Angle Conversion  IU=rad  OU=deg
  Angle Conversion2 : aerolibconvert2/Angle Conversion  IU=rad  OU=deg
  Bounds : Subsystem
  D : Display
  Demux : Demux  Outputs=3
  Derivative : Derivative
  I : Display
  Integrator : Integrator
  Multiply : Gain  Gain=0.001
  Mux : Mux  Inputs=2
  Obs : Subsystem
  P : Display
  Product : Product
  Product1 : Product
  Product2 : Product
  RL Agent : rllib/RL Agent  Agent=agent  ExternalActionAsInput=off  ProvideCumRwd=off  TreatAsDirectFeedthrough=on
  Reward : Subsystem
  Scope : Scope
  Sum2 : Sum  Inputs=+++
  Unit Delay : UnitDelay  SampleTime=-1  HasFrameUpgradeWarning=on
  Controller Output : Outport
  wires:
  Demux/2 -> Product1/1, I/1
  Sum2/1 -> Unit Delay/1, Controller Output/1
  Product2/1 -> Sum2/3
  Derivative/1 -> Product2/2
  Product1/1 -> Sum2/2
  Error/1 -> Product/2, Integrator/1, Derivative/1, Obs/1(Error), Reward/1(Error)
  Product/1 -> Sum2/1
  Integrator/1 -> Product1/2
  Demux/1 -> Product/1, P/1
  Demux/3 -> Product2/1, D/1
  Obs/1(Observations) -> RL Agent/1
  Yaw (Actual)/1 -> Angle Conversion/1, Angle Conversion2/1
  Bounds/1(Boolean) -> RL Agent/3, Reward/2(Boolean)
  Unit Delay/1 -> Reward/3(Delayed Controller Output)
  Reward/1(Reward) -> RL Agent/2
  Mux/1 -> Scope/1
  Yaw (Reference)/1 -> Angle Conversion1/1
  Angle Conversion/1 -> Mux/2
  Angle Conversion1/1 -> Mux/1
  RL Agent/1 -> Multiply/1
  Angle Conversion2/1 -> Bounds/1(Actual Signal)
  Multiply/1 -> Demux/1

== system Drone_PID_rev5_Manual_PID_RL/Controller/Altitude Controller/Z-Controller (Auto-Tune)/Bounds ==
  Actual Signal : Inport
  Compare To Constant : simulink/Logic and Bit Operations/Compare To Constant  relop=<=  const=-15  OutDataTypeStr=boolean
  Compare To Constant1 : simulink/Logic and Bit Operations/Compare To Constant  relop=>  const=0  OutDataTypeStr=boolean
  Logical Operator : Logic  Operator=OR  AllPortsSameDT=off  OutDataTypeStr=boolean
  Boolean : Outport
  wires:
  Logical Operator/1 -> Boolean/1
  Compare To Constant1/1 -> Logical Operator/2
  Actual Signal/1 -> Compare To Constant/1, Compare To Constant1/1
  Compare To Constant/1 -> Logical Operator/1

== system Drone_PID_rev5_Manual_PID_RL/Controller/Altitude Controller/Z-Controller (Auto-Tune)/Obs ==
  Error : Inport
  Discrete Derivative : simulink/Discrete/Discrete Derivative  gainval=1.0  ICPrevScaledInput=0.0  OutMin=[]  OutMax=[]  OutDataType=fixdt(1, 16)  OutScaling=2^-10  DoSatur=off
  Discrete-Time Integrator : DiscreteIntegrator  SampleTime=-1  ICPrevOutput=DiscIntNeverNeededParam  ICPrevScaledInput=DiscIntNeverNeededParam
  Mux : Mux  Inputs=3
  Observations : Outport
  wires:
  Mux/1 -> Observations/1
  Error/1 -> Mux/1, Discrete Derivative/1, Discrete-Time Integrator/1
  Discrete-Time Integrator/1 -> Mux/2
  Discrete Derivative/1 -> Mux/3

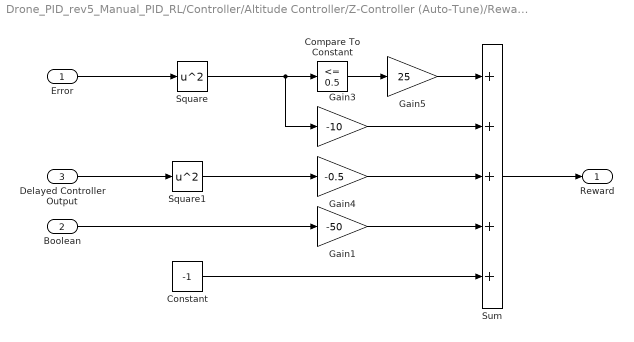
== system Drone_PID_rev5_Manual_PID_RL/Controller/Altitude Controller/Z-Controller (Auto-Tune)/Reward ==
  Error : Inport
  Boolean : Inport  Port=2
  Delayed Controller Output : Inport  Port=3
  Compare To Constant : simulink/Logic and Bit Operations/Compare To Constant  relop=<=  const=0.5  OutDataTypeStr=boolean
  Constant : Constant  Value=-1
  Gain1 : Gain  Gain=-50
  Gain3 : Gain  Gain=-10
  Gain4 : Gain  Gain=-0.5
  Gain5 : Gain  Gain=25
  Square : Math  Operator=square  SaturateOnIntegerOverflow=on
  Square1 : Math  Operator=square  SaturateOnIntegerOverflow=on
  Sum : Sum  Inputs=+++++
  Reward : Outport
  wires:
  Error/1 -> Square/1
  Square/1 -> Gain3/1, Compare To Constant/1
  Boolean/1 -> Gain1/1
  Sum/1 -> Reward/1
  Compare To Constant/1 -> Gain5/1
  Delayed Controller Output/1 -> Square1/1
  Square1/1 -> Gain4/1
  Gain5/1 -> Sum/1
  Gain3/1 -> Sum/2
  Gain4/1 -> Sum/3
  Gain1/1 -> Sum/4
  Constant/1 -> Sum/5

== system Drone_PID_rev5_Manual_PID_RL/Controller/Roll Controller/Roll-Controller (Auto-Tune)/Bounds ==
  Actual Signal : Inport
  Compare To Constant : simulink/Logic and Bit Operations/Compare To Constant  relop=>=  const=15  OutDataTypeStr=boolean
  Compare To Constant1 : simulink/Logic and Bit Operations/Compare To Constant  relop=<  const=0  OutDataTypeStr=boolean
  Logical Operator : Logic  Operator=OR  AllPortsSameDT=off  OutDataTypeStr=boolean
  Boolean : Outport
  wires:
  Logical Operator/1 -> Boolean/1
  Compare To Constant1/1 -> Logical Operator/2
  Actual Signal/1 -> Compare To Constant/1, Compare To Constant1/1
  Compare To Constant/1 -> Logical Operator/1

== system Drone_PID_rev5_Manual_PID_RL/Controller/Roll Controller/Roll-Controller (Auto-Tune)/Obs ==
  Error : Inport
  Discrete Derivative : simulink/Discrete/Discrete Derivative  gainval=1.0  ICPrevScaledInput=0.0  OutMin=[]  OutMax=[]  OutDataType=fixdt(1, 16)  OutScaling=2^-10  DoSatur=off
  Discrete-Time Integrator : DiscreteIntegrator  SampleTime=-1  ICPrevOutput=DiscIntNeverNeededParam  ICPrevScaledInput=DiscIntNeverNeededParam
  Mux : Mux  Inputs=3
  Observations : Outport
  wires:
  Mux/1 -> Observations/1
  Error/1 -> Mux/1, Discrete Derivative/1, Discrete-Time Integrator/1
  Discrete-Time Integrator/1 -> Mux/2
  Discrete Derivative/1 -> Mux/3

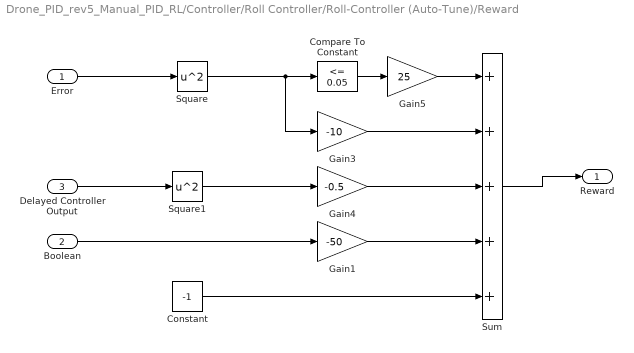
== system Drone_PID_rev5_Manual_PID_RL/Controller/Roll Controller/Roll-Controller (Auto-Tune)/Reward ==
  Error : Inport
  Boolean : Inport  Port=2
  Delayed Controller Output : Inport  Port=3
  Compare To Constant : simulink/Logic and Bit Operations/Compare To Constant  relop=<=  const=0.05  OutDataTypeStr=boolean
  Constant : Constant  Value=-1
  Gain1 : Gain  Gain=-50
  Gain3 : Gain  Gain=-10
  Gain4 : Gain  Gain=-0.5
  Gain5 : Gain  Gain=25
  Square : Math  Operator=square  SaturateOnIntegerOverflow=on
  Square1 : Math  Operator=square  SaturateOnIntegerOverflow=on
  Sum : Sum  Inputs=+++++
  Reward : Outport
  wires:
  Error/1 -> Square/1
  Square/1 -> Gain3/1, Compare To Constant/1
  Boolean/1 -> Gain1/1
  Sum/1 -> Reward/1
  Compare To Constant/1 -> Gain5/1
  Delayed Controller Output/1 -> Square1/1
  Square1/1 -> Gain4/1
  Gain5/1 -> Sum/1
  Gain3/1 -> Sum/2
  Gain4/1 -> Sum/3
  Gain1/1 -> Sum/4
  Constant/1 -> Sum/5

== system Drone_PID_rev5_Manual_PID_RL/Controller/Y Position Controller/Y-Controller (Auto-Tune)/Bounds ==
  Actual Signal : Inport
  Compare To Constant : simulink/Logic and Bit Operations/Compare To Constant  relop=>=  const=15  OutDataTypeStr=boolean
  Compare To Constant1 : simulink/Logic and Bit Operations/Compare To Constant  relop=<  const=0  OutDataTypeStr=boolean
  Logical Operator : Logic  Operator=OR  AllPortsSameDT=off  OutDataTypeStr=boolean
  Boolean : Outport
  wires:
  Logical Operator/1 -> Boolean/1
  Compare To Constant1/1 -> Logical Operator/2
  Actual Signal/1 -> Compare To Constant/1, Compare To Constant1/1
  Compare To Constant/1 -> Logical Operator/1

== system Drone_PID_rev5_Manual_PID_RL/Controller/Y Position Controller/Y-Controller (Auto-Tune)/Obs ==
  Error : Inport
  Discrete Derivative : simulink/Discrete/Discrete Derivative  gainval=1.0  ICPrevScaledInput=0.0  OutMin=[]  OutMax=[]  OutDataType=fixdt(1, 16)  OutScaling=2^-10  DoSatur=off
  Discrete-Time Integrator : DiscreteIntegrator  SampleTime=-1  ICPrevOutput=DiscIntNeverNeededParam  ICPrevScaledInput=DiscIntNeverNeededParam
  Mux : Mux  Inputs=3
  Observations : Outport
  wires:
  Mux/1 -> Observations/1
  Error/1 -> Mux/1, Discrete Derivative/1, Discrete-Time Integrator/1
  Discrete-Time Integrator/1 -> Mux/2
  Discrete Derivative/1 -> Mux/3

== system Drone_PID_rev5_Manual_PID_RL/Controller/Y Position Controller/Y-Controller (Auto-Tune)/Reward ==
  Error : Inport
  Boolean : Inport  Port=2
  Delayed Controller Output : Inport  Port=3
  Compare To Constant : simulink/Logic and Bit Operations/Compare To Constant  relop=<=  const=0.5  OutDataTypeStr=boolean
  Constant : Constant  Value=-1
  Gain1 : Gain  Gain=-50
  Gain3 : Gain  Gain=-10
  Gain4 : Gain  Gain=-0.5
  Gain5 : Gain  Gain=25
  Square : Math  Operator=square  SaturateOnIntegerOverflow=on
  Square1 : Math  Operator=square  SaturateOnIntegerOverflow=on
  Sum : Sum  Inputs=+++++
  Reward : Outport
  wires:
  Error/1 -> Square/1
  Square/1 -> Gain3/1, Compare To Constant/1
  Boolean/1 -> Gain1/1
  Sum/1 -> Reward/1
  Compare To Constant/1 -> Gain5/1
  Delayed Controller Output/1 -> Square1/1
  Square1/1 -> Gain4/1
  Gain5/1 -> Sum/1
  Gain3/1 -> Sum/2
  Gain4/1 -> Sum/3
  Gain1/1 -> Sum/4
  Constant/1 -> Sum/5

== system Drone_PID_rev5_Manual_PID_RL/Controller/Yaw Controller/Yaw-Controller (Auto-Tune)/Bounds ==
  Actual Signal : Inport
  Compare To Constant : simulink/Logic and Bit Operations/Compare To Constant  relop=>=  const=15  OutDataTypeStr=boolean
  Compare To Constant1 : simulink/Logic and Bit Operations/Compare To Constant  relop=<  const=0  OutDataTypeStr=boolean
  Logical Operator : Logic  Operator=OR  AllPortsSameDT=off  OutDataTypeStr=boolean
  Boolean : Outport
  wires:
  Logical Operator/1 -> Boolean/1
  Compare To Constant1/1 -> Logical Operator/2
  Actual Signal/1 -> Compare To Constant/1, Compare To Constant1/1
  Compare To Constant/1 -> Logical Operator/1

== system Drone_PID_rev5_Manual_PID_RL/Controller/Yaw Controller/Yaw-Controller (Auto-Tune)/Obs ==
  Error : Inport
  Discrete Derivative : simulink/Discrete/Discrete Derivative  gainval=1.0  ICPrevScaledInput=0.0  OutMin=[]  OutMax=[]  OutDataType=fixdt(1, 16)  OutScaling=2^-10  DoSatur=off
  Discrete-Time Integrator : DiscreteIntegrator  SampleTime=-1  ICPrevOutput=DiscIntNeverNeededParam  ICPrevScaledInput=DiscIntNeverNeededParam
  Mux : Mux  Inputs=3
  Observations : Outport
  wires:
  Mux/1 -> Observations/1
  Error/1 -> Mux/1, Discrete Derivative/1, Discrete-Time Integrator/1
  Discrete-Time Integrator/1 -> Mux/2
  Discrete Derivative/1 -> Mux/3

== system Drone_PID_rev5_Manual_PID_RL/Controller/Yaw Controller/Yaw-Controller (Auto-Tune)/Reward ==
  Error : Inport
  Boolean : Inport  Port=2
  Delayed Controller Output : Inport  Port=3
  Compare To Constant : simulink/Logic and Bit Operations/Compare To Constant  relop=<=  const=0.05  OutDataTypeStr=boolean
  Constant : Constant  Value=-1
  Gain1 : Gain  Gain=-50
  Gain3 : Gain  Gain=-10
  Gain4 : Gain  Gain=-0.5
  Gain5 : Gain  Gain=25
  Square : Math  Operator=square  SaturateOnIntegerOverflow=on
  Square1 : Math  Operator=square  SaturateOnIntegerOverflow=on
  Sum : Sum  Inputs=+++++
  Reward : Outport
  wires:
  Error/1 -> Square/1
  Square/1 -> Gain3/1, Compare To Constant/1
  Boolean/1 -> Gain1/1
  Sum/1 -> Reward/1
  Compare To Constant/1 -> Gain5/1
  Delayed Controller Output/1 -> Square1/1
  Square1/1 -> Gain4/1
  Gain5/1 -> Sum/1
  Gain3/1 -> Sum/2
  Gain4/1 -> Sum/3
  Gain1/1 -> Sum/4
  Constant/1 -> Sum/5
